simulink library "csu_valvesim_signal_interface_mtv_lib"  (R2014b)
settings: Solver=ode45  StartTime=0.0  StopTime=10.0  RelTol=1e-3
libraries: util_info_lib x1
settings Model: Creator=escrane  LastModifiedBy=mstewart

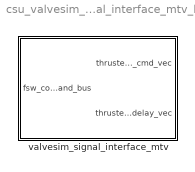
== system csu_valvesim_signal_interface_mtv_lib ==
  valvesim_signal_interface_mtv : Subsystem

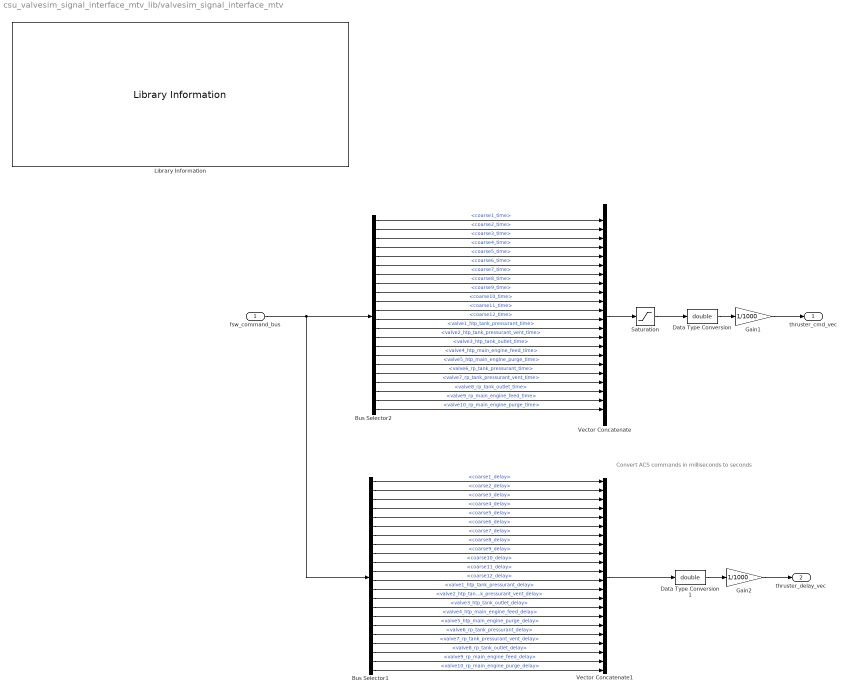
== system csu_valvesim_signal_interface_mtv_lib/valvesim_signal_interface_mtv ==
  note: Convert ACS commands in milliseconds to seconds
  fsw_command_bus : Inport
  Bus Selector1 : BusSelector  OutputSignals=act_mtv_msg.coarse1_delay,act_mtv_msg.coarse2_delay,act_mtv_msg.coarse3_delay,act_mtv_msg.coarse4_delay,act_mtv_msg.coarse5_delay,act_mtv_msg.coarse6_delay,act_mtv_msg.coarse7_delay,act_mtv_msg.coarse8_delay,act_mtv_msg.coarse9_delay,act_mtv_msg.coarse10_delay,act_mtv_msg.coarse11_delay,act_mtv_msg.coarse12_delay,act_mtv_msg.valve1_htp_tank_pressurant_delay,act_mtv_msg.valve2_htp_tank_pressurant_vent_delay,act_mtv_msg.valve3_htp_tank_outlet_delay,act_mtv_msg.valve4_htp_main_engine_feed_delay,act_mtv_msg.valve5_htp_main_engine_purge_delay,act_mtv_msg.valve6_rp_tank_pressurant_delay,act_mtv_msg.valve7_rp_tank_pressurant_vent_delay,act_mtv_msg.valve8_rp_tank_outlet_delay,act_mtv_msg.valve9_rp_main_engine_feed_delay,act_mtv_msg.valve10_rp_main_engine_purge_delay
  Bus Selector2 : BusSelector  OutputSignals=act_mtv_msg.coarse1_time,act_mtv_msg.coarse2_time,act_mtv_msg.coarse3_time,act_mtv_msg.coarse4_time,act_mtv_msg.coarse5_time,act_mtv_msg.coarse6_time,act_mtv_msg.coarse7_time,act_mtv_msg.coarse8_time,act_mtv_msg.coarse9_time,act_mtv_msg.coarse10_time,act_mtv_msg.coarse11_time,act_mtv_msg.coarse12_time,act_mtv_msg.valve1_htp_tank_pressurant_time,act_mtv_msg.valve2_htp_tank_pressurant_vent_time,act_mtv_msg.valve3_htp_tank_outlet_time,act_mtv_msg.valve4_htp_main_engine_feed_time,act_mtv_msg.valve5_htp_main_engine_purge_time,act_mtv_msg.valve6_rp_tank_pressurant_time,act_mtv_msg.valve7_rp_tank_pressurant_vent_time,act_mtv_msg.valve8_rp_tank_outlet_time,act_mtv_msg.valve9_rp_main_engine_feed_time,act_mtv_msg.valve10_rp_main_engine_purge_time
  Data Type Conversion : DataTypeConversion  OutDataTypeStr=double
  Data Type Conversion1 : DataTypeConversion  OutDataTypeStr=double
  Gain1 : Gain  Gain=1/1000  OutDataTypeStr=double
  Gain2 : Gain  Gain=1/1000  OutDataTypeStr=double
  Library Information : util_info_lib/Library Information  owner='NONE'
  Saturation : Saturate  UpperLimit=100  LowerLimit=0
  Vector Concatenate : Concatenate  NumInputs=22
  Vector Concatenate1 : Concatenate  NumInputs=22
  thruster_cmd_vec : Outport
  thruster_delay_vec : Outport  Port=2
  wires:
  Bus Selector1/22 -> Vector Concatenate1/22  "<valve10_rp_main_engine_purge_delay>"
  Bus Selector1/21 -> Vector Concatenate1/21  "<valve9_rp_main_engine_feed_delay>"
  Bus Selector1/20 -> Vector Concatenate1/20  "<valve8_rp_tank_outlet_delay>"
  Bus Selector1/19 -> Vector Concatenate1/19  "<valve7_rp_tank_pressurant_vent_delay>"
  Bus Selector1/18 -> Vector Concatenate1/18  "<valve6_rp_tank_pressurant_delay>"
  Bus Selector1/17 -> Vector Concatenate1/17  "<valve5_htp_main_engine_purge_delay>"
  Bus Selector1/16 -> Vector Concatenate1/16  "<valve4_htp_main_engine_feed_delay>"
  Bus Selector1/15 -> Vector Concatenate1/15  "<valve3_htp_tank_outlet_delay>"
  Bus Selector1/14 -> Vector Concatenate1/14  "<valve2_htp_tank_pressurant_vent_delay>"
  Bus Selector1/13 -> Vector Concatenate1/13  "<valve1_htp_tank_pressurant_delay>"
  Bus Selector2/22 -> Vector Concatenate/22  "<valve10_rp_main_engine_purge_time>"
  Bus Selector2/21 -> Vector Concatenate/21  "<valve9_rp_main_engine_feed_time>"
  Bus Selector2/20 -> Vector Concatenate/20  "<valve8_rp_tank_outlet_time>"
  Bus Selector2/19 -> Vector Concatenate/19  "<valve7_rp_tank_pressurant_vent_time>"
  Bus Selector2/18 -> Vector Concatenate/18  "<valve6_rp_tank_pressurant_time>"
  Bus Selector2/17 -> Vector Concatenate/17  "<valve5_htp_main_engine_purge_time>"
  Bus Selector2/16 -> Vector Concatenate/16  "<valve4_htp_main_engine_feed_time>"
  Bus Selector2/15 -> Vector Concatenate/15  "<valve3_htp_tank_outlet_time>"
  Bus Selector2/14 -> Vector Concatenate/14  "<valve2_htp_tank_pressurant_vent_time>"
  Bus Selector2/13 -> Vector Concatenate/13  "<valve1_htp_tank_pressurant_time>"
  Saturation/1 -> Data Type Conversion/1
  Data Type Conversion/1 -> Gain1/1
  fsw_command_bus/1 -> Bus Selector2/1, Bus Selector1/1
  Vector Concatenate/1 -> Saturation/1
  Gain1/1 -> thruster_cmd_vec/1
  Bus Selector1/2 -> Vector Concatenate1/2  "<coarse2_delay>"
  Bus Selector1/8 -> Vector Concatenate1/8  "<coarse8_delay>"
  Bus Selector1/9 -> Vector Concatenate1/9  "<coarse9_delay>"
  Bus Selector1/4 -> Vector Concatenate1/4  "<coarse4_delay>"
  Bus Selector1/1 -> Vector Concatenate1/1  "<coarse1_delay>"
  Bus Selector1/6 -> Vector Concatenate1/6  "<coarse6_delay>"
  Bus Selector1/12 -> Vector Concatenate1/12  "<coarse12_delay>"
  Bus Selector1/11 -> Vector Concatenate1/11  "<coarse11_delay>"
  Bus Selector1/3 -> Vector Concatenate1/3  "<coarse3_delay>"
  Bus Selector1/10 -> Vector Concatenate1/10  "<coarse10_delay>"
  Bus Selector1/7 -> Vector Concatenate1/7  "<coarse7_delay>"
  Bus Selector1/5 -> Vector Concatenate1/5  "<coarse5_delay>"
  Bus Selector2/1 -> Vector Concatenate/1  "<coarse1_time>"
  Bus Selector2/5 -> Vector Concatenate/5  "<coarse5_time>"
  Bus Selector2/2 -> Vector Concatenate/2  "<coarse2_time>"
  Bus Selector2/3 -> Vector Concatenate/3  "<coarse3_time>"
  Bus Selector2/4 -> Vector Concatenate/4  "<coarse4_time>"
  Bus Selector2/6 -> Vector Concatenate/6  "<coarse6_time>"
  Bus Selector2/7 -> Vector Concatenate/7  "<coarse7_time>"
  Bus Selector2/8 -> Vector Concatenate/8  "<coarse8_time>"
  Bus Selector2/9 -> Vector Concatenate/9  "<coarse9_time>"
  Bus Selector2/12 -> Vector Concatenate/12  "<coarse12_time>"
  Data Type Conversion1/1 -> Gain2/1
  Gain2/1 -> thruster_delay_vec/1
  Bus Selector2/10 -> Vector Concatenate/10  "<coarse10_time>"
  Bus Selector2/11 -> Vector Concatenate/11  "<coarse11_time>"
  Vector Concatenate1/1 -> Data Type Conversion1/1
